simulink model "enable_test2"  (R2017b)
settings: Solver=FixedStepAuto  StartTime=0.0  StopTime=10.0  FixedStep=1.000000  RelTol=1e-3  EnableMultiTasking=on
libraries: simulink x2
settings Model: Creator=hamza  LastModifiedBy=hbourbou
settings DataIOCC: SaveFormat=StructureWithTime
settings OptimizationCC: LifeSpan=inf
settings DebuggingCC: SFUnexpectedBacktrackingDiag=warning  SFNoUnconditionalDefaultTransitionDiag=warning  SFExecutionAtInitializationDiag=none
settings HardwareCC: ProdBitPerSizeT=32  ProdBitPerPtrDiffT=32  ProdWordSize=32  ProdHWDeviceType=Specified
settings CodeAppCC: StateflowObjectComments=on
settings GRTTargetCC: TargetLangStandard=C89/C90 (ANSI)  GeneratePreprocessorConditionals=Disable all
settings ConfigComp: CovMetricSettings=dw  CovHtmlReporting=on  CovSaveCumulativeToWorkspaceVar=on  CovSaveSingleToWorkspaceVar=on  CovExternalEMLEnable=off

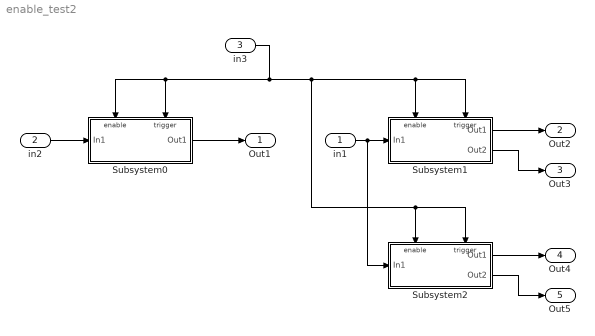
== system enable_test2 ==
  in1 : Inport
  in2 : Inport  Port=2
  in3 : Inport  Port=3  OutDataTypeStr=boolean
  Subsystem0 : Subsystem  TreatAsAtomicUnit=on
  Subsystem1 : Subsystem  TreatAsAtomicUnit=on
  Subsystem2 : Subsystem  TreatAsAtomicUnit=on
  Out1 : Outport
  Out2 : Outport  Port=2
  Out3 : Outport  Port=3
  Out4 : Outport  Port=4
  Out5 : Outport  Port=5
  wires:
  Subsystem0/1(Out1) -> Out1/1
  Subsystem1/1(Out1) -> Out2/1
  in1/1 -> Subsystem2/1(In1), Subsystem1/1(In1)
  in2/1 -> Subsystem0/1(In1)
  Subsystem1/2(Out2) -> Out3/1
  Subsystem2/1(Out1) -> Out4/1
  Subsystem2/2(Out2) -> Out5/1
  in3/1 -> Subsystem1/Enable, Subsystem1/Trigger, Subsystem2/Trigger, Subsystem2/Enable, Subsystem0/Trigger, Subsystem0/Enable

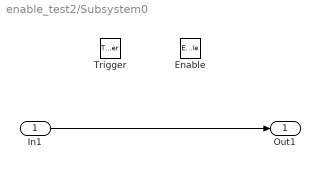
== system enable_test2/Subsystem0 ==
  In1 : Inport
  Enable : EnablePort
  Trigger : TriggerPort  TriggerType=falling  VariantControl=(inherit)
  Out1 : Outport
  wires:
  In1/1 -> Out1/1

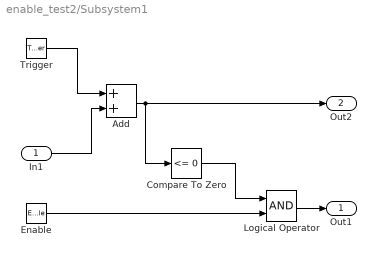
== system enable_test2/Subsystem1 ==
  In1 : Inport
  Enable : EnablePort  ShowOutputPort=on
  Trigger : TriggerPort  TriggerType=either  VariantControl=(inherit)  ShowOutputPort=on
  Add : Sum
  Compare To Zero : simulink/Logic and Bit Operations/Compare To Zero  relop=<=  OutDataTypeStr=boolean
  Logical Operator : Logic  AllPortsSameDT=off  OutDataTypeStr=boolean
  Out1 : Outport
  Out2 : Outport  Port=2
  wires:
  In1/1 -> Add/2
  Trigger/1 -> Add/1
  Add/1 -> Out2/1, Compare To Zero/1
  Enable/1 -> Logical Operator/2
  Logical Operator/1 -> Out1/1
  Compare To Zero/1 -> Logical Operator/1

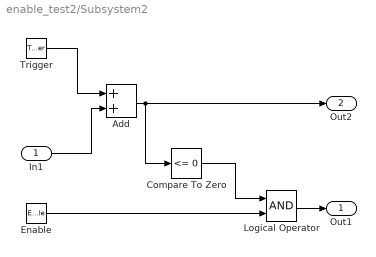
== system enable_test2/Subsystem2 ==
  In1 : Inport
  Enable : EnablePort  StatesWhenEnabling=reset  ShowOutputPort=on
  Trigger : TriggerPort  TriggerType=either  VariantControl=(inherit)  ShowOutputPort=on
  Add : Sum
  Compare To Zero : simulink/Logic and Bit Operations/Compare To Zero  relop=<=  OutDataTypeStr=boolean
  Logical Operator : Logic  AllPortsSameDT=off  OutDataTypeStr=boolean
  Out1 : Outport
  Out2 : Outport  Port=2
  wires:
  In1/1 -> Add/2
  Trigger/1 -> Add/1
  Add/1 -> Out2/1, Compare To Zero/1
  Enable/1 -> Logical Operator/2
  Logical Operator/1 -> Out1/1
  Compare To Zero/1 -> Logical Operator/1
